simulink model "UAV_sync_unknown_gap_sim"  (R2018b)
settings: Solver=ode23tb  StartTime=0.0  StopTime=35  RelTol=1e-3
values from neighbouring files (symbols this model uses):
  Bm = [zeros(6,6); eye(6)]    [UAV_sync_unknown.m]    (also in UAV_sync_unknown_gap.m)
  C_rho = 1.225    [SC42120_UAV_Preconditions.m]
  D0 = [M0 0 0 0 0 0 ... (first row only)    [SC42120_UAV_Preconditions.m]
  Derivative_gain_phi = 50    [SC42120_UAV_Preconditions.m]
  Derivative_gain_psi = 50    [SC42120_UAV_Preconditions.m]
  Derivative_gain_theta = 50    [SC42120_UAV_Preconditions.m]
  Derivative_gain_x = 50    [SC42120_UAV_Preconditions.m]
  Derivative_gain_y = 50    [SC42120_UAV_Preconditions.m]
  Derivative_gain_z = 50    [SC42120_UAV_Preconditions.m]
  G = 9.80665    [SC42120_UAV_Preconditions.m]
  g0 = [0;0;-M0*G;0;0;0]    [SC42120_UAV_Preconditions.m]
  I0 = [0.02 0 -0.01 ... (first row only)    [SC42120_UAV_Preconditions.m]
  I2 = 2*[0.1 0 -0.01 ... (first row only)    [UAV_sync_known.m]    (also in UAV_sync_unknown.m; UAV_sync_unknown_gap.m)
  InitWind = [0;0;0]    [SC42120_UAV_Preconditions.m]
  Kp = diag(P)    [SC42120_UAV_Preconditions.m]
  Kv = diag(V)    [SC42120_UAV_Preconditions.m]
  M0 = 10    [SC42120_UAV_Preconditions.m]
  M1 = 20    [UAV_sync_known.m]    (also in UAV_sync_unknown.m; UAV_sync_unknown_gap.m)
  M2 = 30    [UAV_sync_known.m]    (also in UAV_sync_unknown.m; UAV_sync_unknown_gap.m)
  M3 = 40    [UAV_sync_known.m]    (also in UAV_sync_unknown.m; UAV_sync_unknown_gap.m)
  M4 = 50    [UAV_sync_known.m]    (also in UAV_sync_unknown.m; UAV_sync_unknown_gap.m)
  P = [Proportional_x Proportional_y Proportional_z Proportional_phi Proportional_theta Proportional_psi]    [SC42120_UAV_Preconditions.m]    (also in UAV_sync_unknown.m = lyap(Am',Q); UAV_sync_unknown_gap.m = lyap(Am',Q); drawDATCOMaircraft.m = temparray)
  Proportional_phi = 50    [SC42120_UAV_Preconditions.m]
  Proportional_psi = 50    [SC42120_UAV_Preconditions.m]
  Proportional_theta = 50    [SC42120_UAV_Preconditions.m]
  Proportional_x = 50    [SC42120_UAV_Preconditions.m]
  Proportional_y = 50    [SC42120_UAV_Preconditions.m]
  Proportional_z = 50    [SC42120_UAV_Preconditions.m]
  x_gap = 50    [UAV_sync_unknown_gap.m]
  y_gap = 100    [UAV_sync_unknown_gap.m]
undefined symbols (not defined in the file or in its folder): Aero, APlane, Bxl, C, Ctr, deg, DiscIntNeverNeededParam, F, Guid, Init, Light, MIL, Path, rad, s, Trim, Utility
libraries: aerolibconvert2 x37, sharedutil x20, simulink x15, dspsigops x7, shared6dof x6, aerolibasang x4, simulink_extras x3, aerolibadyn x1, aerolibtransform2 x1, aerolibwind2 x1
(part 6 of 7)

== system UAV_sync_unknown_gap_sim/Node 0/VF Approach/AUTOPILOT/Low-level Controllers/Pitch controller/Coordination offset/tan ==
  In1 : Inport
  Angle Conversion : aerolibconvert2/Angle Conversion  Commented=through  IU=deg  OU=rad
  Angle Conversion1 : aerolibconvert2/Angle Conversion  Commented=through  IU=rad  OU=deg
  Trigonometric Function : Trigonometry  Operator=tan
  Out1 : Outport
  wires:
  In1/1 -> Angle Conversion/1
  Angle Conversion1/1 -> Out1/1
  Angle Conversion/1 -> Trigonometric Function/1
  Trigonometric Function/1 -> Angle Conversion1/1

== system UAV_sync_unknown_gap_sim/Node 0/VF Approach/AUTOPILOT/Low-level Controllers/Pitch controller/Pitch PID/Adjust integrator gain ==
  Constant10 : Constant  Value=0.15
  Ctr.Pitch.PTCH2SRV_TCONST : Gain  Gain=Ctr.Pitch.PTCH2SRV_TCONST
  MinMax : MinMax  Function=max  Inputs=2
  K_I rate : Outport
  wires:
  ? -> MinMax/1
  Ctr.Pitch.PTCH2SRV_TCONST/1 -> K_I rate/1  "ki_rate"
  Constant10/1 -> MinMax/2
  MinMax/1 -> Ctr.Pitch.PTCH2SRV_TCONST/1

== system UAV_sync_unknown_gap_sim/Node 0/VF Approach/AUTOPILOT/Low-level Controllers/Pitch controller/Pitch PID/Anti-windup ==
  u : Inport
  y : Inport  Port=2
  If : If  IfExpression=u1 < -45  ElseIfExpressions=u1 > 45
  If Action Subsystem : Subsystem  TreatAsAtomicUnit=on
  If Action Subsystem1 : Subsystem  TreatAsAtomicUnit=on
  If Action Subsystem2 : Subsystem  TreatAsAtomicUnit=on
  Merge : Merge  Inputs=3
  y_int : Outport
  wires:
  If Action Subsystem1/1(Out1) -> Merge/2
  Merge/1 -> y_int/1
  If Action Subsystem2/1(Out1) -> Merge/3
  y/1 -> If/1
  If Action Subsystem/1(Out1) -> Merge/1
  u/1 -> If Action Subsystem/1(In1), If Action Subsystem1/1(In1), If Action Subsystem2/1(In1)
  If/2 -> If Action Subsystem1/Action
  If/1 -> If Action Subsystem/Action
  If/3 -> If Action Subsystem2/Action

== system UAV_sync_unknown_gap_sim/Node 0/VF Approach/AUTOPILOT/Low-level Controllers/Pitch controller/Pitch PID/Subsystem ==
  In1 : Inport
  Meas_roll_angle : Inport  Port=2
  Meas_pitch_rate : Inport  Port=3  Unit=deg/s
  +-45 : Saturate  UpperLimit=45  LowerLimit=-45
  Abs : Abs
  Abs1 : Abs
  Gain : Gain  Gain=-1
  If : If  IfExpression=u1 > 90
  If Action Subsystem : Subsystem  TreatAsAtomicUnit=on
  If Action Subsystem1 : Subsystem  TreatAsAtomicUnit=on
  If Action Subsystem2 : Subsystem  TreatAsAtomicUnit=on
  If Action Subsystem3 : Subsystem  TreatAsAtomicUnit=on
  If1 : If  NumInputs=2  IfExpression=u1 >84 & u2 < 70
  Merge : Merge
  Merge1 : Merge
  Out1 : Outport
  wires:
  If Action Subsystem3/1(Out1) -> Merge1/2
  Abs/1 -> If Action Subsystem/1(In1), If Action Subsystem1/1(In1), If/1
  Meas_pitch_rate/1 -> Abs1/1
  If/1 -> If Action Subsystem/Action
  Merge/1 -> If Action Subsystem2/1(In1), If1/1  "roll wrapped"
  If Action Subsystem2/1(Out1) -> Merge1/1
  +-45/1 -> Gain/1
  If1/2 -> If Action Subsystem3/Action
  Abs1/1 -> If1/2
  If Action Subsystem1/1(Out1) -> Merge/2
  Meas_roll_angle/1 -> Abs/1
  If1/1 -> If Action Subsystem2/Action
  In1/1 -> If Action Subsystem3/1(In1), If Action Subsystem2/2(In2)
  Gain/1 -> Out1/1
  If Action Subsystem/1(Out1) -> Merge/1
  If/2 -> If Action Subsystem1/Action
  Merge1/1 -> [lastO], +-45/1

== system UAV_sync_unknown_gap_sim/Node 0/VF Approach/AUTOPILOT/Low-level Controllers/Pitch controller/TRASH/If Action Subsystem ==
  Action Port : ActionPort
  Constant : Constant  Value=0
  Out1 : Outport
  wires:
  Constant/1 -> Out1/1

== system UAV_sync_unknown_gap_sim/Node 0/VF Approach/AUTOPILOT/Low-level Controllers/Pitch controller/TRASH/If Action Subsystem1 ==
  pitch : Inport
  bank : Inport  Port=2
  Va : Inport  Port=3
  Action Port : ActionPort
  Abs : Abs
  Constant : Constant  Value=C.g
  Constant1 : Constant  Value=APlane.EAS2TAS
  Constant2 : Constant  Value=APlane.airspeed_min
  Constant3 : Constant  Value=Ctr.Pitch.PTCH2SRV_RLL
  MinMax : MinMax  Function=max  Inputs=2
  Product : Product  Inputs=***
  Product1 : Product  Inputs=*/**
  Product2 : Product  Inputs=**
  bank1 : InportShadow  Port=2
  cosd : Subsystem
  sind : Subsystem
  tand : Subsystem
  Out1 : Outport
  wires:
  Product/1 -> Out1/1
  Abs/1 -> Product/2
  Constant/1 -> Product1/1
  MinMax/1 -> Product1/2
  Constant1/1 -> Product2/2
  Va/1 -> Product2/1
  Product2/1 -> MinMax/1
  Constant2/1 -> MinMax/2
  cosd/1(Out1) -> Product/1
  bank/1 -> tand/1(In1)
  bank1/1 -> sind/1(In1)
  Product1/1 -> Abs/1
  pitch/1 -> cosd/1(In1)
  tand/1(Out1) -> Product1/3
  sind/1(Out1) -> Product1/4
  Constant3/1 -> Product/3

== system UAV_sync_unknown_gap_sim/Node 0/VF Approach/AUTOPILOT/Low-level Controllers/Pitch controller/TRASH/Parameters mixer1 ==
  note: 9
  note: 8
  note: 7
  note: 6
  note: 5
  note: 4
  note: 3
  note: 2
  note: 1
  Constant : Constant  Value=Ctr.Pitch.PTCH2SRV_I
  Constant1 : Constant  Value=Ctr.Pitch.PTCH2SRV_D
  Constant2 : Constant  Value=Ctr.Pitch.PTCH2SRV_FF
  Constant3 : Constant  Value=Ctr.Pitch.PTCH2SRV_P
  Constant4 : Constant  Value=APlane.roll_limit
  Constant5 : Constant  Value=Ctr.Pitch.PTCH2SRV_IMAX
  Constant6 : Constant  Value=APlane.airspeed_min
  Constant7 : Constant  Value=APlane.EAS2TAS
  Constant8 : Constant  Value=Ctr.Pitch.PTCH2SRV_TCONST
  Mux : Mux  Inputs=9
  parameters : Outport
  wires:
  Mux/1 -> parameters/1
  Constant8/1 -> Mux/1
  Constant3/1 -> Mux/2
  Constant/1 -> Mux/3
  Constant1/1 -> Mux/4
  Constant5/1 -> Mux/5
  Constant2/1 -> Mux/6
  Constant6/1 -> Mux/7
  Constant7/1 -> Mux/8
  Constant4/1 -> Mux/9

== system UAV_sync_unknown_gap_sim/Node 0/VF Approach/AUTOPILOT/Low-level Controllers/Pitch controller/TRASH/Parameters mixer2 ==
  Constant2 : Constant  Value=Ctr.Pitch.PTCH2SRV_RLL
  Constant3 : Constant  Value=C.g
  Constant5 : Constant  Value=APlane.EAS2TAS
  Constant6 : Constant  Value=APlane.airspeed_min
  Mux1 : Mux
  parameters_roll_comp : Outport
  wires:
  Constant6/1 -> Mux1/4
  Constant5/1 -> Mux1/3
  Mux1/1 -> parameters_roll_comp/1
  Constant3/1 -> Mux1/2
  Constant2/1 -> Mux1/1

== system UAV_sync_unknown_gap_sim/Node 0/VF Approach/AUTOPILOT/Low-level Controllers/Roll controller/Roll Rate Controller/Anti-windup ==
  y : Inport
  u : Inport  Port=2
  If : If  IfExpression=u1 < -45  ElseIfExpressions=u1 > 45
  If Action Subsystem : Subsystem  TreatAsAtomicUnit=on
  If Action Subsystem1 : Subsystem  TreatAsAtomicUnit=on
  If Action Subsystem2 : Subsystem  TreatAsAtomicUnit=on
  Merge : Merge  Inputs=3
  y_int : Outport
  wires:
  If Action Subsystem1/1(Out1) -> Merge/2
  Merge/1 -> y_int/1
  If Action Subsystem2/1(Out1) -> Merge/3
  y/1 -> If/1
  If Action Subsystem/1(Out1) -> Merge/1
  u/1 -> If Action Subsystem/1(In1), If Action Subsystem1/1(In1), If Action Subsystem2/1(In1)
  If/2 -> If Action Subsystem1/Action
  If/1 -> If Action Subsystem/Action
  If/3 -> If Action Subsystem2/Action

== system UAV_sync_unknown_gap_sim/Node 0/VF Approach/AUTOPILOT/Low-level Controllers/Roll controller/Roll Rate Controller/K_FF (real feedforward) ==
  Constant5 : Constant  Value=Ctr.Roll.RLL2SRV_FF
  Constant6 : Constant  Value=APlane.EAS2TAS
  Product1 : Product  Inputs=*/
  Out1 : Outport
  wires:
  Product1/1 -> Out1/1  "k_ff"
  Constant6/1 -> Product1/2
  Constant5/1 -> Product1/1

== system UAV_sync_unknown_gap_sim/Node 0/VF Approach/AUTOPILOT/Low-level Controllers/Roll controller/Roll Rate Controller/K_P (feedforward) ==
  Constant : Constant  Value=APlane.EAS2TAS
  Constant2 : Constant  Value=0
  Constant7 : Constant  Value=Ctr.Roll.K_P
  MinMax : MinMax  Function=max  Inputs=2
  Product : Product  Inputs=*/
  Out1 : Outport
  wires:
  Constant2/1 -> MinMax/2
  Constant7/1 -> MinMax/1
  MinMax/1 -> Product/1
  Product/1 -> Out1/1  "kp_ff"
  Constant/1 -> Product/2

== system UAV_sync_unknown_gap_sim/Node 0/VF Approach/BIXLER DYNAMICS/RUBBISH BIN/Straight Line/SL.controller/Param. Mixer ==
  Constant1 : Constant  Value=Guid.SL.chi_inf
  Constant2 : Constant  Value=Guid.Est.alpha
  Constant3 : Constant  Value=Guid.SL.kk
  Constant4 : Constant  Value=Guid.SL.eps
  Constant5 : Constant  Value=Guid.SL.k
  Mux : Mux  Inputs=5
  param : Outport
  wires:
  Constant2/1 -> Mux/5  "alpha"
  Constant3/1 -> Mux/4  "kk"
  Constant5/1 -> Mux/3  "k"
  Constant1/1 -> Mux/2  "chi_inf"
  Constant4/1 -> Mux/1  "eps"
  Mux/1 -> param/1

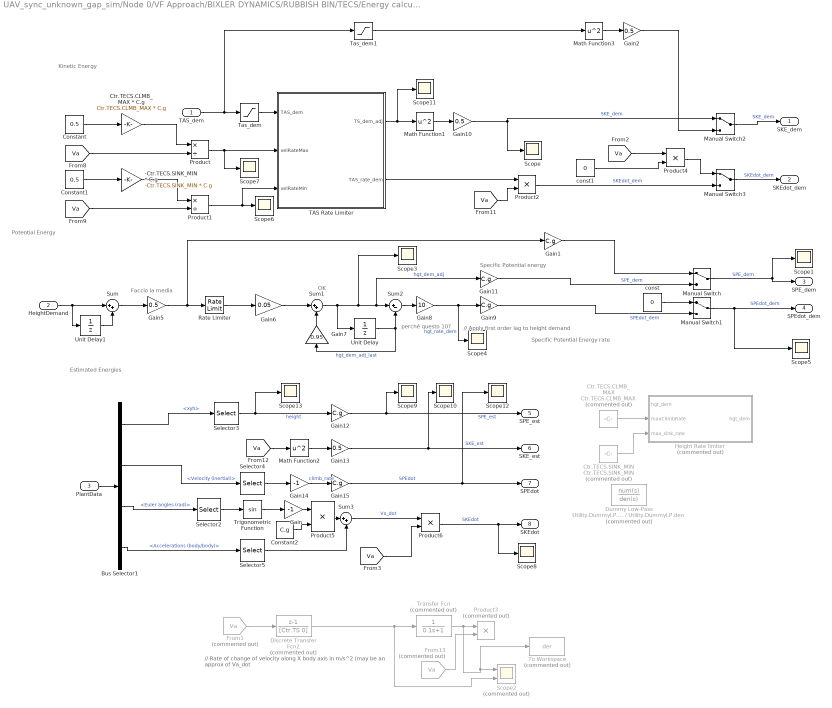
== system UAV_sync_unknown_gap_sim/Node 0/VF Approach/BIXLER DYNAMICS/RUBBISH BIN/TECS/Energy calculations/Calculate energies ==
  note: Estimated Energies
  note: Potential Energy
  note: Kinetic Energy
  note: // Apply first order lag to height demand
  note: perché questo 10?
  note: Specific Potential Energy rate
  note: Specific Potential energy
  note: OK
  note: Faccio la media
  note: // Rate of change of velocity along X body axis in m/s^2
      | (may be an approx of Va_dot
  TAS_dem : Inport
  HeightDemand : Inport  Port=2
  PlantData : Inport  Port=3
  -Ctr.TECS.SINK_MIN * C.g : Gain  Gain=-Ctr.TECS.SINK_MIN * C.g
  Bus Selector1 : BusSelector  OutputSignals=xyh,Velocity (inertial),Euler angles (rad),Accelerations (body/body)
  Constant : Constant  Value=0.5
  Constant1 : Constant  Value=0.5
  Constant2 : Constant  Value=C.g
  Ctr.TECS.CLMB_MAX : Constant  Commented=on  Value=Ctr.TECS.CLMB_MAX
  Ctr.TECS.CLMB_MAX * C.g : Gain  Gain=Ctr.TECS.CLMB_MAX * C.g
  Ctr.TECS.SINK_MIN : Constant  Commented=on  Value=Ctr.TECS.SINK_MIN
  Discrete Transfer Fcn2 : DiscreteTransferFcn  Commented=on  Numerator=[1 -1]  Denominator=[Ctr.TS 0]  SampleTime=Ctr.TS
  Dummy Low-Pass : TransferFcn  Commented=on  Numerator=Utility.DummyLP.num  Denominator=Utility.DummyLP.den
  From1 : From  Commented=on  GotoTag=Va  TagVisibility=global
  From13 : From  Commented=on  GotoTag=Va  TagVisibility=global
  Gain : Gain  Gain=-1
  Gain{1,9,11..12,15} (5 alike) : Gain  Gain=C.g
  Gain{2,5,10,13} (4 alike) : Gain  Gain=0.5
  Gain14 : Gain  Gain=-1
  Gain6 : Gain  Gain=0.05
  Gain7 : Gain  Gain=0.95
  Gain8 : Gain  Gain=10
  Height Rate limiter : MATLAB Function  Commented=on  TreatAsAtomicUnit=on
  Manual Switch{,1..3} (4 alike) : ManualSwitch
  Math Function1 : Math  Operator=square  SaturateOnIntegerOverflow=on
  Math Function2 : Math  Operator=square  SaturateOnIntegerOverflow=on
  Math Function3 : Math  Operator=square  SaturateOnIntegerOverflow=on
  Product : Product  Inputs=*/
  Product1 : Product  Inputs=*/
  Product{2,4..6} (4 alike) : Product
  Product3 : Product  Commented=on
  Rate Limiter : RateLimiter  RisingSlewLimit=Ctr.TECS.CLMB_MAX  FallingSlewLimit=-Ctr.TECS.SINK_MIN  SampleTimeMode=inherited
  Scope{,1,3..13} (13 alike) : Scope
  Scope2 : Scope  Commented=on  NumInputPorts=2
  Selector2 : Selector  InputPortWidth=3  IndexOptions=Index vector (dialog)  Indices=2  OutputSizes=1
  Selector3 : Selector  InputPortWidth=3  IndexOptions=Index vector (dialog)  Indices=3  OutputSizes=1
  Selector4 : Selector  InputPortWidth=3  IndexOptions=Index vector (dialog)  Indices=3  OutputSizes=1
  Selector5 : Selector  InputPortWidth=3  IndexOptions=Index vector (dialog)  Indices=1  OutputSizes=1
  Sum : Sum  Inputs=|++
  Sum1 : Sum  Inputs=|++
  Sum2 : Sum  Inputs=|+-
  Sum3 : Sum  Inputs=|++
  TAS Rate Limiter : MATLAB Function  TreatAsAtomicUnit=on
  Tas_dem : Saturate  UpperLimit=35  LowerLimit=6
  Tas_dem1 : Saturate  UpperLimit=35  LowerLimit=6
  To Workspace : ToWorkspace  Commented=on  VariableName=der  SampleTime=-1
  Transfer Fcn : TransferFcn  Commented=on  Numerator=1  Denominator=[0.1 1]
  Trigonometric Function : Trigonometry
  Unit Delay : UnitDelay  SampleTime=Ctr.TS
  Unit Delay1 : UnitDelay  SampleTime=Ctr.TS
  const : Constant  Value=0
  const1 : Constant  Value=0
  SKE_dem : Outport
  SKEdot_dem : Outport  Port=2
  SPE_dem : Outport  Port=3
  SPEdot_dem : Outport  Port=4
  SPE_est : Outport  Port=5
  SKE_est : Outport  Port=6
  SPEdot : Outport  Port=7
  SKEdot : Outport  Port=8
  wires:
  Gain5/1 -> Gain1/1, Rate Limiter/1
  Gain8/1 -> Scope4/1, Gain9/1  "hgt_rate_dem"
  Gain6/1 -> Sum1/1
  Sum/1 -> Gain5/1
  Ctr.TECS.CLMB_MAX/1 -> Height Rate limiter/2(maxClimbRate)
  Ctr.TECS.SINK_MIN/1 -> Height Rate limiter/3(max_sink_rate)
  -Ctr.TECS.SINK_MIN * C.g/1 -> Product1/1
  Ctr.TECS.CLMB_MAX * C.g/1 -> Product/1
  Manual Switch/1 -> SPE_dem/1, Scope1/1  "SPE_dem"
  Sum2/1 -> Gain8/1
  Unit Delay/1 -> Gain7/1, Sum2/2  "hgt_dem_adj_last"
  Product2/1 -> Manual Switch3/2  "SKEdot_dem"
  Sum1/1 -> Unit Delay/1, Scope3/1, Gain11/1, Sum2/1  "hgt_dem_adj"
  Manual Switch1/1 -> Scope5/1, SPEdot_dem/1  "SPEdot_dem"
  [Va] -> Product2/2
  Gain12/1 -> Scope9/1, SPE_est/1  "SPE_est"
  Gain14/1 -> Gain15/1  "climb_rate"
  Gain13/1 -> Scope10/1, SKE_est/1  "SKE_est"
  TAS Rate Limiter/1(TS_dem_adj) -> Scope11/1, Math Function1/1
  Math Function2/1 -> Gain13/1
  TAS Rate Limiter/2(TAS_rate_dem) -> Product2/1
  Gain10/1 -> Manual Switch2/1, Scope/1  "SKE_dem"
  Math Function1/1 -> Gain10/1
  Selector3/1 -> Scope13/1, Gain12/1  "height"
  [Va] -> Math Function2/1
  Constant1/1 -> -Ctr.TECS.SINK_MIN * C.g/1
  Product1/1 -> Scope6/1, TAS Rate Limiter/3(velRateMin)
  Product/1 -> Scope7/1, TAS Rate Limiter/2(velRateMax)
  Gain7/1 -> Sum1/2
  Constant/1 -> Ctr.TECS.CLMB_MAX * C.g/1
  TAS_dem/1 -> Tas_dem1/1, Tas_dem/1
  HeightDemand/1 -> Unit Delay1/1, Sum/1
  Gain15/1 -> Scope12/1, SPEdot/1  "SPEdot"
  PlantData/1 -> Bus Selector1/1
  Bus Selector1/1 -> Selector3/1  "<xyh>"
  Bus Selector1/2 -> Selector4/1  "<Velocity (inertial)>"
  [Va] -> Product/2
  Selector4/1 -> Gain14/1
  [Va] -> Product1/2
  Rate Limiter/1 -> Gain6/1
  Unit Delay1/1 -> Sum/2
  Gain11/1 -> Manual Switch/2  "SPE_dem"
  Gain9/1 -> Manual Switch1/2  "SPEdot_dem"
  Gain1/1 -> Manual Switch/1
  Manual Switch2/1 -> SKE_dem/1  "SKE_dem"
  Math Function3/1 -> Gain2/1
  Gain2/1 -> Manual Switch2/2
  const1/1 -> Product4/2
  Tas_dem/1 -> TAS Rate Limiter/1(TAS_dem)
  [Va] -> Product4/1
  Product4/1 -> Manual Switch3/1
  Manual Switch3/1 -> SKEdot_dem/1  "SKEdot_dem"
  From13/1 -> Product3/2
  Product6/1 -> Scope8/1, SKEdot/1  "SKEdot"
  From1/1 -> Discrete Transfer Fcn2/1
  Discrete Transfer Fcn2/1 -> Transfer Fcn/1, Scope2/2
  Transfer Fcn/1 -> To Workspace/1, Scope2/1, Product3/1
  Bus Selector1/3 -> Selector2/1  "<Euler angles (rad)>"
  Sum3/1 -> Product6/1  "Vx_dot"
  [Va] -> Product6/2
  Selector2/1 -> Trigonometric Function/1
  Constant2/1 -> Product5/2
  Bus Selector1/4 -> Selector5/1  "<Accelerations (body/body)>"
  Product5/1 -> Sum3/1
  Selector5/1 -> Sum3/2
  Gain/1 -> Product5/1
  Trigonometric Function/1 -> Gain/1
  Tas_dem1/1 -> Math Function3/1
  const/1 -> Manual Switch1/1

== system UAV_sync_unknown_gap_sim/Node 0/VF Approach/BIXLER DYNAMICS/RUBBISH BIN/TECS/PITCH/DT1 ==
  Clock1 : Clock
  Memory : Memory  InheritSampleTime=on
  Sum : Sum  Inputs=|+-
  DT : Outport
  wires:
  Memory/1 -> Sum/2
  Sum/1 -> DT/1
  Clock1/1 -> Memory/1, Sum/1

== system UAV_sync_unknown_gap_sim/Node 0/VF Approach/BIXLER DYNAMICS/RUBBISH BIN/TECS/PITCH/Limiter ==
  integSEB_input : Inport
  PITCHmaxf : Inport  Port=2
  PITCHminf : Inport  Port=3
  pitch_dem : Inport  Port=4
  If : If  NumInputs=3  IfExpression=u1 > u2  ElseIfExpressions=u1 < u3
  If Action Subsystem : Subsystem  TreatAsAtomicUnit=on
  If Action Subsystem1 : Subsystem  TreatAsAtomicUnit=on
  If Action Subsystem2 : Subsystem  TreatAsAtomicUnit=on
  Merge : Merge  Inputs=3
  PITCHmaxf_1 : InportShadow  Port=2
  PITCHminf_1 : InportShadow  Port=3
  pitch_dem_1 : InportShadow  Port=4
  SEB_in_lim : Outport
  wires:
  If Action Subsystem1/1(Out1) -> Merge/3
  If Action Subsystem/1(Out1) -> Merge/1
  If Action Subsystem2/1(Out1) -> Merge/2
  PITCHminf_1/1 -> If Action Subsystem1/2(PITCHminf)
  integSEB_input/1 -> If/1, If Action Subsystem1/1(integSEB_input), If Action Subsystem2/1(integSEB_input), If Action Subsystem/1(integSEB_input)
  pitch_dem_1/1 -> If Action Subsystem1/3(pitch_dem)
  PITCHmaxf_1/1 -> If Action Subsystem/2(PITCHmaxf)
  If/3 -> If Action Subsystem2/Action
  PITCHmaxf/1 -> If/2
  Merge/1 -> SEB_in_lim/1
  PITCHminf/1 -> If/3
  pitch_dem/1 -> If Action Subsystem/3(pitch_dem)
  If/1 -> If Action Subsystem/Action
  If/2 -> If Action Subsystem1/Action

== system UAV_sync_unknown_gap_sim/Node 0/VF Approach/BIXLER DYNAMICS/RUBBISH BIN/TECS/PITCH/integSEB ==
  temp : Inport
  gainInv : Inport  Port=2
  PITCHminf : Inport  Port=3
  PITCHmaxf : Inport  Port=4
  integSEB_delta : Inport  Port=5
  Constant : Constant  Value=0.0783
  Constant1 : Constant  Value=0.0783
  Gain : Gain  Gain=0.1
  Gain1 : Gain  Gain=-0.1
  Product : Product
  Product1 : Product
  Saturation Dynamic : simulink/Discontinuities/Saturation Dynamic  OutMin=[]  OutMax=[]  OutDataTypeStr=Inherit: Same as second input  OutDataType=fixdt(1, 16)  OutScaling=2^-10  DoSatur=off
  Sum : Sum  Inputs=|+-
  Sum1 : Sum  Inputs=|+-
  Sum2 : Sum  Inputs=|++
  Sum3 : Sum  Inputs=-+|
  Sum4 : Sum  Inputs=|+-
  gainInv_1 : InportShadow  Port=2
  "integSEB_min " : Outport
  "IntegSEB_delta " : Outport  Port=2
  integSEB_max : Outport  Port=3
  wires:
  PITCHminf/1 -> Sum/1
  Product/1 -> Sum1/1
  Constant1/1 -> Sum2/2
  Sum3/1 -> integSEB_max/1, [integSEB_max]
  PITCHmaxf/1 -> Sum2/1
  Sum2/1 -> Product1/2
  gainInv_1/1 -> Product1/1
  Constant/1 -> Sum/2
  integSEB_delta/1 -> Saturation Dynamic/2
  Sum/1 -> Product/2
  Sum1/1 -> "integSEB_min "/1, [integSEB_min]
  temp/1 -> Sum3/1, Sum1/2
  [integSEB_range] -> Gain1/1
  Gain1/1 -> Saturation Dynamic/3
  Saturation Dynamic/1 -> "IntegSEB_delta "/1
  Sum4/1 -> [integSEB_range]
  [integSEB_min] -> Sum4/2
  [integSEB_max] -> Sum4/1
  [integSEB_range] -> Gain/1
  Gain/1 -> Saturation Dynamic/1
  gainInv/1 -> Product/1
  Product1/1 -> Sum3/2

== system UAV_sync_unknown_gap_sim/Node 0/VF Approach/BIXLER DYNAMICS/RUBBISH BIN/TECS/PITCH/timeConstant() ==
  Constant1 : Constant  Value=0.1
  Constant5 : Constant  Value=Ctr.TECS.TIME_CONST
  MinMax : MinMax  Function=max  Inputs=2
  timeConstant : Outport
  wires:
  MinMax/1 -> timeConstant/1
  Constant1/1 -> MinMax/2
  Constant5/1 -> MinMax/1

== system UAV_sync_unknown_gap_sim/Node 0/VF Approach/BIXLER DYNAMICS/RUBBISH BIN/TECS/PITCH/timeConstant()1 ==
  Constant1 : Constant  Value=0.1
  Constant5 : Constant  Value=Ctr.TECS.TIME_CONST
  MinMax : MinMax  Function=max  Inputs=2
  timeConstant : Outport
  wires:
  MinMax/1 -> timeConstant/1
  Constant1/1 -> MinMax/2
  Constant5/1 -> MinMax/1

== system UAV_sync_unknown_gap_sim/Node 0/VF Approach/BIXLER DYNAMICS/RUBBISH BIN/TECS/PITCH1/DT1 ==
  Clock1 : Clock
  Memory : Memory  InheritSampleTime=on
  Sum : Sum  Inputs=|+-
  DT : Outport
  wires:
  Memory/1 -> Sum/2
  Sum/1 -> DT/1
  Clock1/1 -> Memory/1, Sum/1

== system UAV_sync_unknown_gap_sim/Node 0/VF Approach/BIXLER DYNAMICS/RUBBISH BIN/TECS/PITCH1/Limiter ==
  integSEB_input : Inport
  PITCHmaxf : Inport  Port=2
  PITCHminf : Inport  Port=3
  pitch_dem : Inport  Port=4
  If : If  NumInputs=3  IfExpression=u1 > u2  ElseIfExpressions=u1 < u3
  If Action Subsystem : Subsystem  TreatAsAtomicUnit=on
  If Action Subsystem1 : Subsystem  TreatAsAtomicUnit=on
  If Action Subsystem2 : Subsystem  TreatAsAtomicUnit=on
  Merge : Merge  Inputs=3
  PITCHmaxf_1 : InportShadow  Port=2
  PITCHminf_1 : InportShadow  Port=3
  pitch_dem_1 : InportShadow  Port=4
  y : Outport
  wires:
  If Action Subsystem1/1(Out1) -> Merge/3
  If Action Subsystem/1(Out1) -> Merge/1
  If Action Subsystem2/1(Out1) -> Merge/2
  PITCHminf_1/1 -> If Action Subsystem1/2(PITCHminf)
  integSEB_input/1 -> If/1, If Action Subsystem1/1(integSEB_input), If Action Subsystem2/1(integSEB_input), If Action Subsystem/1(integSEB_input)
  pitch_dem_1/1 -> If Action Subsystem1/3(pitch_dem)
  PITCHmaxf_1/1 -> If Action Subsystem/2(PITCHmaxf)
  If/3 -> If Action Subsystem2/Action
  PITCHmaxf/1 -> If/2
  Merge/1 -> y/1
  PITCHminf/1 -> If/3
  pitch_dem/1 -> If Action Subsystem/3(pitch_dem)
  If/1 -> If Action Subsystem/Action
  If/2 -> If Action Subsystem1/Action

== system UAV_sync_unknown_gap_sim/Node 0/VF Approach/BIXLER DYNAMICS/RUBBISH BIN/TECS/PITCH1/integSEB ==
  temp : Inport
  gainInv : Inport  Port=2
  PITCHminf : Inport  Port=3
  PITCHmaxf : Inport  Port=4
  integSEB_delta : Inport  Port=5
  Constant : Constant  Value=0.0783
  Constant1 : Constant  Value=0.0783
  Gain : Gain  Gain=0.1
  Gain1 : Gain  Gain=-0.1
  Product : Product
  Product1 : Product
  Saturation Dynamic : simulink/Discontinuities/Saturation Dynamic  OutMin=[]  OutMax=[]  OutDataTypeStr=Inherit: Same as second input  OutDataType=fixdt(1, 16)  OutScaling=2^-10  DoSatur=off
  Sum{,1,3..4} (4 alike) : Sum  Inputs=|+-
  Sum2 : Sum  Inputs=|++
  gainInv_1 : InportShadow  Port=2
  temp_1 : InportShadow
  "IntegSEB_delta " : Outport
  "integSEB_min " : Outport  Port=2
  integSEB_max : Outport  Port=3
  wires:
  PITCHminf/1 -> Sum/1
  Product/1 -> Sum1/1
  Constant1/1 -> Sum2/2
  Sum3/1 -> integSEB_max/1, [integSEB_max]
  PITCHmaxf/1 -> Sum2/1
  Sum2/1 -> Product1/2
  Product1/1 -> Sum3/1
  gainInv_1/1 -> Product1/1
  temp_1/1 -> Sum3/2
  Constant/1 -> Sum/2
  integSEB_delta/1 -> Saturation Dynamic/2
  Sum/1 -> Product/2
  Sum1/1 -> "integSEB_min "/1, [integSEB_min]
  temp/1 -> Sum1/2
  [integSEB_range] -> Gain1/1
  Gain1/1 -> Saturation Dynamic/3
  Saturation Dynamic/1 -> "IntegSEB_delta "/1
  Sum4/1 -> [integSEB_range]
  [integSEB_min] -> Sum4/2
  [integSEB_max] -> Sum4/1
  [integSEB_range] -> Gain/1
  Gain/1 -> Saturation Dynamic/1
  gainInv/1 -> Product/1

== system UAV_sync_unknown_gap_sim/Node 0/VF Approach/BIXLER DYNAMICS/RUBBISH BIN/TECS/PITCH1/timeConstant() ==
  Constant1 : Constant  Value=0.1
  Constant5 : Constant  Value=Ctr.TECS.TIME_CONST
  MinMax : MinMax  Function=max  Inputs=2
  timeConstant : Outport
  wires:
  MinMax/1 -> timeConstant/1
  Constant1/1 -> MinMax/2
  Constant5/1 -> MinMax/1

== system UAV_sync_unknown_gap_sim/Node 0/VF Approach/BIXLER DYNAMICS/RUBBISH BIN/TECS/PITCH1/timeConstant()1 ==
  Constant1 : Constant  Value=0.1
  Constant5 : Constant  Value=Ctr.TECS.TIME_CONST
  MinMax : MinMax  Function=max  Inputs=2
  timeConstant : Outport
  wires:
  MinMax/1 -> timeConstant/1
  Constant1/1 -> MinMax/2
  Constant5/1 -> MinMax/1

== system UAV_sync_unknown_gap_sim/Node 0/VF Approach/BIXLER DYNAMICS/Vehicle Airframe/Aerodynamics/Aerodynamic Coefficients/Forces ==
  note: CL
  note: Cy
  note: CD
  note: f_y is already in the body frame
  alpha_k : Inport
  alpha_f : Inport  Port=2
  CD interpolation : Interpolation_n-D  NumberOfTableDimensions=1  Table=Aero.CD_Basic  RemoveProtectionIndex=on  InternalRulePriority=Speed
      settings: InputPortMap=u0,u1
  CL interpolation : Interpolation_n-D  NumberOfTableDimensions=1  Table=Aero.CL_Basic  RemoveProtectionIndex=on  InternalRulePriority=Speed
      settings: InputPortMap=u0,u1
  CYp Interpolation : Interpolation_n-D  NumberOfTableDimensions=1  Table=Aero.Cy_RollRate  RemoveProtectionIndex=on  InternalRulePriority=Speed
      settings: InputPortMap=u0,u1
  Constant1 : Constant  Value=Aero.CL_PitchRate
  Constant6 : Constant  Value=Aero.Cy_Beta
  Divide1 : Product  Inputs=**/
  Divide3 : Product  Inputs=**
  Divide4 : Product  Inputs=**/
  Gain10 : Gain  Gain=2
  Gain2 : Gain  Gain=Bxl.c
  Gain3 : Gain  Gain=2
  Gain9 : Gain  Gain=Bxl.b
  Sum1 : Sum  Inputs=|++
  Sum3 : Sum  Inputs=++|
  CD : Outport
  Cy : Outport  Port=2
  CL : Outport  Port=3
  wires:
  Gain2/1 -> Divide1/1
  Constant1/1 -> Gain2/1
  Gain3/1 -> Divide1/3
  [Va] -> Gain3/1
  [qRad] -> Divide1/2  "q=pitch rate"
  Divide1/1 -> Sum1/2
  [pRad] -> Divide4/2  "q=roll rate"
  [Va] -> Gain10/1
  Gain9/1 -> Divide4/1
  Gain10/1 -> Divide4/3
  Sum3/1 -> Cy/1  "Cy"
  CL interpolation/1 -> Sum1/1  "CL(alpha)"
  CYp Interpolation/1 -> Gain9/1
  alpha_k/1 -> CL interpolation/1, CYp Interpolation/1, CD interpolation/1
  alpha_f/1 -> CL interpolation/2, CYp Interpolation/2, CD interpolation/2
  Divide4/1 -> Sum3/2
  CD interpolation/1 -> CD/1  "CD(alpha)"
  Sum1/1 -> CL/1  "CL"
  [BetaRad] -> Divide3/2
  Constant6/1 -> Divide3/1
  Divide3/1 -> Sum3/1

== system UAV_sync_unknown_gap_sim/Node 0/VF Approach/BIXLER DYNAMICS/Vehicle Airframe/Aerodynamics/Aerodynamic Coefficients/Moments ==
  note: Cn
  note: Cl
  note: Cm
  note: Moments already in the body frame
  alpha_k : Inport
  alpha_f : Inport  Port=2
  Clb Interpolation : Interpolation_n-D  NumberOfTableDimensions=1  Table=Aero.Cl_Beta  RemoveProtectionIndex=on  InternalRulePriority=Speed
      settings: InputPortMap=u0,u1
  Clp Interpolation : Interpolation_n-D  NumberOfTableDimensions=1  Table=Aero.Cl_RollRate  RemoveProtectionIndex=on  InternalRulePriority=Speed
      settings: InputPortMap=u0,u1
  Clr Interpolation : Interpolation_n-D  NumberOfTableDimensions=1  Table=Aero.Cl_YawRate  RemoveProtectionIndex=on  InternalRulePriority=Speed
      settings: InputPortMap=u0,u1
  Cm_Basic Interpolation : Interpolation_n-D  NumberOfTableDimensions=1  Table=Aero.Cm_Basic  RemoveProtectionIndex=on  InternalRulePriority=Speed
      settings: InputPortMap=u0,u1
  Cnp : Interpolation_n-D  NumberOfTableDimensions=1  Table=Aero.Cn_RollRate  RemoveProtectionIndex=on  InternalRulePriority=Speed
      settings: InputPortMap=u0,u1
  Cnr : Interpolation_n-D  NumberOfTableDimensions=1  Table=Aero.Cn_YawRate  RemoveProtectionIndex=on  InternalRulePriority=Speed
      settings: InputPortMap=u0,u1
  Constant1 : Constant  Value=0
  Constant2 : Constant  Value=Aero.Cm_PitchRate
  Constant4 : Constant  Value=0
  Constant5 : Constant  Value=Aero.Cn_Beta
  Divide1 : Product  Inputs=**
  Divide3 : Product  Inputs=**
  Divide{4..7,9} (5 alike) : Product  Inputs=**/
  Gain{1,3..4,7,15} (5 alike) : Gain  Gain=2
  Gain{2,5,8,13} (4 alike) : Gain  Gain=Bxl.b
  Gain14 : Gain  Gain=Bxl.c
  Manual Switch2 : ManualSwitch
  Manual Switch3 : ManualSwitch
  Sum{1..2,4..5} (4 alike) : Sum  Inputs=|++
  Sum3 : Sum  Inputs=++|
  Cl : Outport
  Cm : Outport  Port=2
  Cn : Outport  Port=3
  wires:
  alpha_k/1 -> Cnr/1, Cnp/1, Cm_Basic Interpolation/1, Clr Interpolation/1, Clp Interpolation/1, Clb Interpolation/1
  alpha_f/1 -> Cnr/2, Cnp/2, Cm_Basic Interpolation/2, Clr Interpolation/2, Clp Interpolation/2, Clb Interpolation/2
  [Va] -> Gain3/1
  Divide9/1 -> Sum1/2
  Sum1/1 -> Sum3/2
  Gain1/1 -> Divide9/3
  [Va] -> Gain1/1
  Gain2/1 -> Divide9/1
  [rRad] -> Divide9/2  "r=yaw rate"
  Cnp/1 -> Gain8/1
  [pRad] -> Divide4/2  "p=roll rate"
  Sum3/1 -> Cn/1  "Cn"
  Gain8/1 -> Divide4/1
  Gain3/1 -> Divide4/3
  Cnr/1 -> Gain2/1
  Divide3/1 -> Sum2/1
  Clb Interpolation/1 -> Divide3/1
  Gain7/1 -> Divide6/3
  [Va] -> Gain4/1
  Gain4/1 -> Divide5/3
  Sum4/1 -> Cl/1  "Cl"
  Gain5/1 -> Divide5/1
  Gain13/1 -> Divide6/1
  Clp Interpolation/1 -> Gain5/1
  [BetaRad] -> Divide3/2
  [Va] -> Gain7/1
  Clr Interpolation/1 -> Gain13/1
  Divide6/1 -> Manual Switch2/1
  [pRad] -> Divide5/2  "p=roll rate"
  Sum2/1 -> Sum4/1
  [rRad] -> Divide6/2  "r=yaw rate"
  [qRad] -> Divide7/2  "q=pitch rate"
  Gain15/1 -> Divide7/3
  Gain14/1 -> Divide7/1
  Sum5/1 -> Cm/1  "Cm"
  Constant2/1 -> Gain14/1
  Cm_Basic Interpolation/1 -> Sum5/1
  [Va] -> Gain15/1
  Divide7/1 -> Sum5/2
  Divide1/1 -> Sum3/1
  [BetaRad] -> Divide1/2
  Constant5/1 -> Divide1/1
  Divide4/1 -> Sum1/1
  Constant4/1 -> Manual Switch3/2
  Divide5/1 -> Manual Switch3/1
  Manual Switch3/1 -> Sum2/2
  Manual Switch2/1 -> Sum4/2
  Constant1/1 -> Manual Switch2/2

== system UAV_sync_unknown_gap_sim/Node 0/VF Approach/BIXLER DYNAMICS/Vehicle Airframe/Aerodynamics/ControlIncrements/Ailerons ==
  alpha_k : Inport
  alpha_f : Inport  Port=2
  DeltaAil : Inport  Port=3
  Cl_ail Interpolation : Interpolation_n-D  NumberOfTableDimensions=1  Table=Aero.Cl_ail  RemoveProtectionIndex=on  InternalRulePriority=Speed
      settings: InputPortMap=u0,u1
  Cn_ail Interpolation : Interpolation_n-D  Table=Aero.Cn_ail  InternalRulePriority=Speed
  DeltaAil. : PreLookup  BreakpointsData=Aero.delta_ail_vector  BeginIndexSearchUsingPreviousIndexResult=on  ExtrapMethod=Linear  RemoveProtectionInput=on
  Cn_ail : Outport
  Cl_ail : Outport  Port=2
  wires:
  DeltaAil/1 -> DeltaAil./1
  Cn_ail Interpolation/1 -> Cn_ail/1
  Cl_ail Interpolation/1 -> Cl_ail/1
  alpha_f/1 -> Cn_ail Interpolation/2
  DeltaAil./2 -> Cl_ail Interpolation/2, Cn_ail Interpolation/4
  DeltaAil./1 -> Cl_ail Interpolation/1, Cn_ail Interpolation/3
  alpha_k/1 -> Cn_ail Interpolation/1

== system UAV_sync_unknown_gap_sim/Node 0/VF Approach/BIXLER DYNAMICS/Vehicle Airframe/Aerodynamics/ControlIncrements/Elevator ==
  alpha_k : Inport
  alpha_f : Inport  Port=2
  DeltaElev : Inport  Port=3
  CD_elev Interpolation : Interpolation_n-D  Table=Aero.CD_elev  RemoveProtectionIndex=on  InternalRulePriority=Speed
  DeltaElev Interpolation : PreLookup  BreakpointsData=Aero.delta_ail_vector  BeginIndexSearchUsingPreviousIndexResult=on  ExtrapMethod=Linear  RemoveProtectionInput=on
  Gain : Gain  Gain=Aero.CL_elev
  Gain1 : Gain  Gain=Aero.Cm_elev
  Scope : Scope
  Scope1 : Scope
  CD_elev : Outport
  CL_elev : Outport  Port=2
  Cm_elev : Outport  Port=3
  wires:
  Gain1/1 -> Scope1/1, Cm_elev/1
  DeltaElev/1 -> DeltaElev Interpolation/1, Gain1/1, Gain/1
  alpha_k/1 -> CD_elev Interpolation/1
  DeltaElev Interpolation/1 -> CD_elev Interpolation/3
  DeltaElev Interpolation/2 -> CD_elev Interpolation/4
  alpha_f/1 -> CD_elev Interpolation/2
  CD_elev Interpolation/1 -> Scope/1, CD_elev/1
  Gain/1 -> CL_elev/1

== system UAV_sync_unknown_gap_sim/Node 0/VF Approach/BIXLER DYNAMICS/Vehicle Airframe/Aerodynamics/ControlIncrements/Rudder ==
  note: Change of sign to match with the convention.
      | The coefficients are taken from a report of the Bixler 2 flight.
  deltaRudd : Inport
  Gain : Gain  Gain=-1
  Gain1 : Gain  Gain=Aero.Cy_rudd
  Gain2 : Gain  Gain=Aero.Cn_rudd
  Gain3 : Gain  Gain=Aero.Cl_rudd
  Gain4 : Gain  Gain=-1
  Cy_rudd : Outport
  Cl_rudd : Outport  Port=2
  Cn_rudd : Outport  Port=3
  wires:
  Gain3/1 -> Gain4/1
  Gain1/1 -> Gain/1
  deltaRudd/1 -> Gain1/1, Gain3/1, Gain2/1
  Gain2/1 -> Cn_rudd/1
  Gain4/1 -> Cl_rudd/1
  Gain/1 -> Cy_rudd/1

== system UAV_sync_unknown_gap_sim/Node 0/VF Approach/AUTOPILOT/Low-level Controllers/Pitch controller/Pitch PID/Anti-windup/If Action Subsystem ==
  In1 : Inport
  Action Port : ActionPort  ActionType=then
  Constant : Constant  Value=0
  MinMax : MinMax  Function=max  Inputs=2
  Out1 : Outport
  wires:
  In1/1 -> MinMax/1
  Constant/1 -> MinMax/2
  MinMax/1 -> Out1/1

== system UAV_sync_unknown_gap_sim/Node 0/VF Approach/AUTOPILOT/Low-level Controllers/Pitch controller/Pitch PID/Anti-windup/If Action Subsystem1 ==
  In1 : Inport
  Action Port : ActionPort  ActionType=elseif
  Constant : Constant  Value=0
  MinMax : MinMax  Inputs=2
  Out1 : Outport
  wires:
  In1/1 -> MinMax/1
  Constant/1 -> MinMax/2
  MinMax/1 -> Out1/1

== system UAV_sync_unknown_gap_sim/Node 0/VF Approach/AUTOPILOT/Low-level Controllers/Pitch controller/Pitch PID/Anti-windup/If Action Subsystem2 ==
  In1 : Inport
  Action Port : ActionPort  ActionType=else
  Out1 : Outport
  wires:
  In1/1 -> Out1/1

== system UAV_sync_unknown_gap_sim/Node 0/VF Approach/AUTOPILOT/Low-level Controllers/Pitch controller/Pitch PID/Subsystem/If Action Subsystem ==
  In1 : Inport
  Action Port : ActionPort
  Constant : Constant  Value=180
  Sum : Sum  Inputs=|+-
  Out1 : Outport
  wires:
  In1/1 -> Sum/2
  Constant/1 -> Sum/1
  Sum/1 -> Out1/1

== system UAV_sync_unknown_gap_sim/Node 0/VF Approach/AUTOPILOT/Low-level Controllers/Pitch controller/Pitch PID/Subsystem/If Action Subsystem1 ==
  In1 : Inport
  Action Port : ActionPort
  Out1 : Outport
  wires:
  In1/1 -> Out1/1

== system UAV_sync_unknown_gap_sim/Node 0/VF Approach/AUTOPILOT/Low-level Controllers/Pitch controller/Pitch PID/Subsystem/If Action Subsystem2 ==
  In1 : Inport
  In2 : Inport  Port=2
  Action Port : ActionPort
  Fcn : Fcn  Expr=1- ((u(1)-(APlane.roll_limit+5))/(90-APlane.roll_limit))
  Product7 : Product
  Out1 : Outport
  wires:
  In1/1 -> Fcn/1
  Fcn/1 -> Product7/1
  Product7/1 -> Out1/1
  In2/1 -> Product7/2

== system UAV_sync_unknown_gap_sim/Node 0/VF Approach/AUTOPILOT/Low-level Controllers/Pitch controller/Pitch PID/Subsystem/If Action Subsystem3 ==
  In1 : Inport
  Action Port : ActionPort
  Out1 : Outport
  wires:
  In1/1 -> Out1/1

== system UAV_sync_unknown_gap_sim/Node 0/VF Approach/AUTOPILOT/Low-level Controllers/Pitch controller/TRASH/If Action Subsystem1/cosd ==
  In1 : Inport
  Angle Conversion : aerolibconvert2/Angle Conversion  IU=deg  OU=rad
  Angle Conversion1 : aerolibconvert2/Angle Conversion  IU=rad  OU=deg
  Trigonometric Function : Trigonometry  Operator=cos
  Out1 : Outport
  wires:
  Trigonometric Function/1 -> Angle Conversion1/1
  Angle Conversion/1 -> Trigonometric Function/1
  Angle Conversion1/1 -> Out1/1
  In1/1 -> Angle Conversion/1

== system UAV_sync_unknown_gap_sim/Node 0/VF Approach/AUTOPILOT/Low-level Controllers/Pitch controller/TRASH/If Action Subsystem1/sind ==
  In1 : Inport
  Angle Conversion : aerolibconvert2/Angle Conversion  IU=deg  OU=rad
  Angle Conversion1 : aerolibconvert2/Angle Conversion  IU=rad  OU=deg
  Trigonometric Function : Trigonometry
  Out1 : Outport
  wires:
  Trigonometric Function/1 -> Angle Conversion1/1
  Angle Conversion/1 -> Trigonometric Function/1
  Angle Conversion1/1 -> Out1/1
  In1/1 -> Angle Conversion/1

== system UAV_sync_unknown_gap_sim/Node 0/VF Approach/AUTOPILOT/Low-level Controllers/Pitch controller/TRASH/If Action Subsystem1/tand ==
  In1 : Inport
  Angle Conversion : aerolibconvert2/Angle Conversion  IU=deg  OU=rad
  Angle Conversion1 : aerolibconvert2/Angle Conversion  IU=rad  OU=deg
  Trigonometric Function : Trigonometry  Operator=tan
  Out1 : Outport
  wires:
  In1/1 -> Angle Conversion/1
  Angle Conversion1/1 -> Out1/1
  Angle Conversion/1 -> Trigonometric Function/1
  Trigonometric Function/1 -> Angle Conversion1/1

== system UAV_sync_unknown_gap_sim/Node 0/VF Approach/AUTOPILOT/Low-level Controllers/Roll controller/Roll Rate Controller/Anti-windup/If Action Subsystem ==
  In1 : Inport
  Action Port : ActionPort  ActionType=then
  Constant : Constant  Value=0
  MinMax : MinMax  Function=max  Inputs=2
  Out1 : Outport
  wires:
  In1/1 -> MinMax/1
  Constant/1 -> MinMax/2
  MinMax/1 -> Out1/1

== system UAV_sync_unknown_gap_sim/Node 0/VF Approach/AUTOPILOT/Low-level Controllers/Roll controller/Roll Rate Controller/Anti-windup/If Action Subsystem1 ==
  In1 : Inport
  Action Port : ActionPort  ActionType=elseif
  Constant : Constant  Value=0
  MinMax : MinMax  Inputs=2
  Out1 : Outport
  wires:
  In1/1 -> MinMax/1
  Constant/1 -> MinMax/2
  MinMax/1 -> Out1/1

== system UAV_sync_unknown_gap_sim/Node 0/VF Approach/AUTOPILOT/Low-level Controllers/Roll controller/Roll Rate Controller/Anti-windup/If Action Subsystem2 ==
  In1 : Inport
  Action Port : ActionPort  ActionType=else
  Out1 : Outport
  wires:
  In1/1 -> Out1/1

== system UAV_sync_unknown_gap_sim/Node 0/VF Approach/BIXLER DYNAMICS/RUBBISH BIN/TECS/PITCH/Limiter/If Action Subsystem ==
  integSEB_input : Inport
  PITCHmaxf : Inport  Port=2
  pitch_dem : Inport  Port=3
  Action Port : ActionPort
  MinMax : MinMax
  Mux : Mux  Inputs=2
  Sum : Sum  Inputs=|+-
  Out1 : Outport
  wires:
  integSEB_input/1 -> Mux/1
  MinMax/1 -> Out1/1
  PITCHmaxf/1 -> Sum/1
  Sum/1 -> Mux/2
  Mux/1 -> MinMax/1
  pitch_dem/1 -> Sum/2

== system UAV_sync_unknown_gap_sim/Node 0/VF Approach/BIXLER DYNAMICS/RUBBISH BIN/TECS/PITCH/Limiter/If Action Subsystem1 ==
  integSEB_input : Inport
  PITCHminf : Inport  Port=2
  pitch_dem : Inport  Port=3
  Action Port : ActionPort
  MinMax : MinMax  Function=max
  Mux : Mux  Inputs=2
  Sum : Sum  Inputs=|+-
  Out1 : Outport
  wires:
  integSEB_input/1 -> Mux/1
  MinMax/1 -> Out1/1
  PITCHminf/1 -> Sum/1
  pitch_dem/1 -> Sum/2
  Sum/1 -> Mux/2
  Mux/1 -> MinMax/1

== system UAV_sync_unknown_gap_sim/Node 0/VF Approach/BIXLER DYNAMICS/RUBBISH BIN/TECS/PITCH/Limiter/If Action Subsystem2 ==
  integSEB_input : Inport
  Action Port : ActionPort
  Out1 : Outport
  wires:
  integSEB_input/1 -> Out1/1

== system UAV_sync_unknown_gap_sim/Node 0/VF Approach/BIXLER DYNAMICS/RUBBISH BIN/TECS/PITCH1/Limiter/If Action Subsystem ==
  integSEB_input : Inport
  PITCHmaxf : Inport  Port=2
  pitch_dem : Inport  Port=3
  Action Port : ActionPort
  MinMax : MinMax
  Mux : Mux  Inputs=2
  Sum : Sum  Inputs=|+-
  Out1 : Outport
  wires:
  integSEB_input/1 -> Mux/1
  MinMax/1 -> Out1/1
  PITCHmaxf/1 -> Sum/1
  Sum/1 -> Mux/2
  Mux/1 -> MinMax/1
  pitch_dem/1 -> Sum/2

== system UAV_sync_unknown_gap_sim/Node 0/VF Approach/BIXLER DYNAMICS/RUBBISH BIN/TECS/PITCH1/Limiter/If Action Subsystem1 ==
  integSEB_input : Inport
  PITCHminf : Inport  Port=2
  pitch_dem : Inport  Port=3
  Action Port : ActionPort
  MinMax : MinMax  Function=max
  Mux : Mux  Inputs=2
  Sum : Sum  Inputs=|+-
  Out1 : Outport
  wires:
  integSEB_input/1 -> Mux/1
  MinMax/1 -> Out1/1
  PITCHminf/1 -> Sum/1
  pitch_dem/1 -> Sum/2
  Sum/1 -> Mux/2
  Mux/1 -> MinMax/1

== system UAV_sync_unknown_gap_sim/Node 0/VF Approach/BIXLER DYNAMICS/RUBBISH BIN/TECS/PITCH1/Limiter/If Action Subsystem2 ==
  integSEB_input : Inport
  Action Port : ActionPort
  Out1 : Outport
  wires:
  integSEB_input/1 -> Out1/1

== matlab function UAV_sync_unknown_gap_sim/Node 0/VF Approach/BIXLER DYNAMICS/RUBBISH BIN/Orbit/Loiter Controller/Beard Version ==
  data: chi input; chi_c output; chi_d input; d input; Vg input; gamma input; param input
function chi_c  = OrbitController(chi, chi_d, d, Vg, gamma, param)

%%
k = param(1);
kk = param(2);
epsi = param(3);
r = param(4);
j = param(5);
alpha = param(6);

%%
chi_tilde = chi-chi_d;
lt = chi_tilde/epsi;

if abs(lt) <=1
    term = lt;
else
    term = sign(lt);
end

d_tilde = d-r;
beta = k/(1+(k*d_tilde)^2);

err = (chi-gamma);

term2 = Vg /(alpha*d)*sin(err) + j*beta/alpha*Vg*cos(err);

term3 = -kk/alpha*term;

chi_c = chi + term2 + term3;

== matlab function UAV_sync_unknown_gap_sim/Node 0/VF Approach/AUTOPILOT/Low-level Controllers/Pitch controller/TRASH/Pitch_PID_MATLAB_Fcn ==
  data: desired_rate input; meas_pitch_rate input; out output; meas_roll_angle input; scaler input; aspeed input; time input; parteInt output; parteDer output; parteFF output; parteP output; parameters input
function [out, parteInt, parteDer, parteFF, parteP] = pitch_rate_controller...
    (desired_rate, meas_pitch_rate, meas_roll_angle, scaler, aspeed, time, ... % inputs
    parameters) % parameters
%%

gainstau = parameters(1);
gainsP = parameters(2);
gainsI = parameters(3);
gainsD = parameters(4);
gainsimax = parameters(5);
gainsFF = parameters(6);
airspeed_min = parameters(7);
eas2tas = parameters(8);
roll_limit = parameters(9);

persistent last_t;
persistent last_out;
persistent pidInfoI;

if isempty(last_t)
    last_t = 0;
end

if isempty(pidInfoI)
    pidInfoI = 0;
end

if isempty(last_out)
    last_out = 0;
end

if time==0
    last_t = 0;
    last_out=0;
    pidInfoI=0;
end

%% Start of code

tnow = time;
dt = tnow - last_t;

if (last_t == 0 || dt > 1)
    dt = 0;
end

last_t = tnow;

delta_time = dt; % * 0.001; Because the microcontroller gives [ms] - REMOVED

achieved_rate = meas_pitch_rate;
rate_error = rad2deg((desired_rate - achieved_rate) * scaler);

if gainsI > 0
    k_I = gainsI;
        if (gainsFF == 0)
    %                     /*
    %               if the user hasn't set a direct FF then assume they are
    %               not doing sophisticated tuning. Set a minimum I value of
    %               0.15 to ensure that the time constant for trimming in
    %               pitch is not too long. We have had a lot of user issues
    %               with very small I value leading to very slow pitch
    %               trimming, which causes a lot of problems for TECS. A
    %               value of 0.15 is still quite small, but a lot better
    %               than what many users are running.
    %              */
            k_I = max(k_I, 0.15);
        end
    ki_rate = k_I * gainstau;
    %     only integrate if gain and time step are positive and airspeed above min value.
    if (dt > 0 && aspeed > 0.5*airspeed_min)
        integrator_delta = rate_error * ki_rate * delta_time * scaler;
        if last_out < -45
            %              prevent the integrator from increasing if surface defln demand is above the upper limit
            integrator_delta = max(integrator_delta, 0);
        elseif last_out > 45
            %             prevent the integrator from decreasing if surface defln demand  is below the lower limit
            integrator_delta = min(integrator_delta, 0);
        end
        pidInfoI = pidInfoI + integrator_delta;
    end
else
    pidInfoI = 0;
end

intLimScaled = gainsimax * 0.01;
pidInfoI = constrain_value(pidInfoI, -intLimScaled, intLimScaled);


% get ESTIMATED to TRUE airspeed ratio (assuming 1, as in
% Airspeed_calibration.cpp)

% Calculate equivalent gains so that values for K_P and K_I can be taken across from the old PID law
% No conversion is required for K_D
kp_ff = max((gainsP - gainsI * gainstau) * gainstau  - gainsD , 0) / eas2tas;
k_ff = gainsFF / eas2tas;

% Calculate the demanded control surface deflection
% Note the scaler is applied again. We want a 1/speed scaler applied to the feed-forward
% path, but want a 1/speed^2 scaler applied to the rate error path.
% This is because acceleration scales with speed^2, but rate scales with speed.
pidInfoD = rate_error * gainsD * scaler;
pidInfoP = desired_rate * kp_ff * scaler;
pidInfoFF = desired_rate * k_ff * scaler;
last_out = pidInfoFF + pidInfoP + pidInfoD;
% pidInfodesired = desired_rate;
last_out = last_out + pidInfoI;

% when we are past the users defined roll limit for the
% aircraft our priority should be to bring the aircraft back
% within the roll limit. Using elevator for pitch control at
% large roll angles is ineffective, and can be counter
% productive as it induces earth-frame yaw which can reduce
% the ability to roll. We linearly reduce elevator input when
% beyond the configured roll limit, reducing to zero at 90
% degrees
roll_wrapped = rad2deg(abs(meas_roll_angle));

if roll_wrapped > 90
    roll_wrapped = 180-roll_wrapped;
end
% 
% if (roll_wrapped>roll_limit+5 && roll_limit<85 && abs(meas_pitch_rate) < 70)
%     roll_prop = (roll_wrapped - (roll_limit+5) / (90-roll_limit));
%     last_out = last_out * (1 - roll_prop);
% end

out = constrain_value(last_out * 100, -4500, 4500);

parteInt = pidInfoI;
parteDer = pidInfoD;
parteFF = pidInfoFF;
parteP = pidInfoP;

== matlab function UAV_sync_unknown_gap_sim/Node 0/VF Approach/BIXLER DYNAMICS/RUBBISH BIN/Straight Line/Vg Estimator/SL_Estimator ==
  data: chi input; chi_d input; chi_q input; e input; Vg_hat input; Vg_hat_dot output size=1; param input; e output; f1 output; f2 output; Vg input
function [Vg_hat_dot, e, f1, f2]...
    = estimator (chi, chi_d, chi_q, e, Vg_hat, param, Vg)
%  feedback, der, term2, last_term,diff_chi, diff_2,
%estimator of Vg'
%% Parameters
y_int = param(1);
W = param(2);
Va = param(3);
epsi = param(4);
phiw = param(5);
chi_inf = param(6);
k = param(7);
kk=param(8);
Gamma = param(9);
sigma = param(10);

%% Law

rho = y_int^2/pi^2;   % Positive scale factor used to weight the terms so that y and chi are similar in magnitude

diff_chi = chi-chi_d; % Error of course angle

term =diff_chi/epsi;
if abs(term)<=1
    sat=term;
else
    sat=sign(term);
end

% % derivative of Vg' over x'
der = W*sin(phiw-chi)+(Va^2-W^2*(sin(phiw-chi))^2)^(-0.5)*W^2*sin(phiw-chi)*cos(phiw-chi); % partial derivative of Vg' over chi'
% 
% % Vg2_hat_dot =-i*Gamma*rho*diff_chi*chi_inf*2/pi*(k*(sin(chi2)-a*cos(chi2)))/(1+(k*(e))^2)+der*(i*chi_inf*2/pi*(k*(sin(chi2)-a*cos(chi2)))/(1+(k*(e))^2)*Vg2_hat-kk*sat);
term2 = (-1*chi_inf*2/pi*(k*sin(chi - chi_q))/(1+(k*(e))^2)*Vg_hat);
last_term = -1*kk*sat;
f2 = (sin(chi - chi_q));
f1 =  k/(1+(k*e)^2)*Gamma*rho*diff_chi*chi_inf*2/pi;

alpha = 0.4578;

% if Vg_hat - Vg > 0.5
%     sigma = (Vg_hat - Vg);
% else
%     sigma = 0;
% end
Gamma = 5;
Vg_hat_dot = Gamma/alpha*rho*diff_chi*chi_inf*2/pi*(k*(sin(chi-chi_q)))/(1+(k*(e))^2)...
    - sigma* Gamma * Vg_hat +...
     1*der*(term2/alpha +last_term);



end

== matlab function UAV_sync_unknown_gap_sim/Node 0/VF Approach/AUTOPILOT/Low-level Controllers/Pitch controller/TRASH/Coordination_offset_MATLAB_Fcn ==
  data: bank_angle input; rate_offset output; meas_pitch_angle input; aspeed input; parameters input; inverted output
function [rate_offset, inverted] = coord_rate_offset(bank_angle, meas_pitch_angle, aspeed, parameters)

param = [  parameters(1), parameters(2), parameters(3), parameters(4) ];
[rate_offset, inverted] = get_coordination_rate(bank_angle, meas_pitch_angle, aspeed, param);

== matlab function UAV_sync_unknown_gap_sim/Node 0/VF Approach/BIXLER DYNAMICS/RUBBISH BIN/TECS/Energy calculations/Calculate energies/TAS Rate Limiter ==
  data: TS_dem_adj output; TAS_dem input; TAS_rate_dem output; velRateMax input; velRateMin input
function [TS_dem_adj, TAS_rate_dem] = RateLimiter (TAS_dem, velRateMax, velRateMin)

persistent TAS_dem_adj
persistent TAS_dem_last

TASmin = 6;
TASmax = 35;

if isempty(TAS_dem_adj)
    TAS_dem_adj = 0;
end

if isempty(TAS_dem_last)
    TAS_dem_last = 0;
end


% Apply rate limit
if ((TAS_dem - TAS_dem_adj) > (velRateMax * 0.1))
    TAS_dem_adj = TAS_dem_adj + velRateMax * 0.1;
    TAS_rate_dem = velRateMax;
elseif ((TAS_dem - TAS_dem_adj) < (velRateMin * 0.1))
    TAS_dem_adj = TAS_dem_adj + velRateMin * 0.1;
    TAS_rate_dem = velRateMin;
else
    TAS_dem_adj = TAS_dem;
    TAS_rate_dem = (TAS_dem - TAS_dem_last) / 0.1;
end
%     Constrain speed demand again to protect against bad values on initialisation.
TAS_dem_adj = constrain_value(TAS_dem_adj, TASmin, TASmax);

TS_dem_adj = TAS_dem_adj; % Output 
TAS_dem_last = TAS_dem;

== matlab function UAV_sync_unknown_gap_sim/Node 0/VF Approach/BIXLER DYNAMICS/RUBBISH BIN/TECS/PITCH1/Integrator ==
  data: integSEB_delta input; y output; integSEB_min input; integSEB_max input
function y = fcn(integSEB_delta, integSEB_min, integSEB_max)

persistent integSEB_state

if isempty(integSEB_state)
    integSEB_state = 0;
end

integSEB_state = constrain_value(integSEB_state + integSEB_delta, integSEB_min, integSEB_max);

y = integSEB_state;

== matlab function UAV_sync_unknown_gap_sim/Node 0/VF Approach/BIXLER DYNAMICS/RUBBISH BIN/Straight Line/Compute crosstrack error/Xtrack error ==
  data: x input; chi_q output; y input; chi input; slope input; origin input; epy output
function [chi_q, epy]= fcn(x, y, chi, slope, origin)

chi_q = atan2(slope(2),slope(1));    % Course of the straight line [rad]
 
while chi_q - chi < -pi
    chi_q = chi_q + 2*pi;
end
while chi_q - chi > pi
    chi_q = chi_q - 2*pi;
end

epy = -sin(chi_q)*(x-origin(1)) + cos(chi_q)*(y-origin(2));
